simulink model "RCmodel"  (Simulink 7.0)
settings: Solver=ode3  StartTime=0.0  StopTime=0.02  RelTol=1e-3
InitFcn:
  | init;
values from neighbouring files (symbols this model uses):
  C = 1e-6    (= 1e-06)    [initRC.m]
  R = 1000    [initRC.m]
  T0 = tau/5    (= 0.0002)    [initRC.m]
  tau = R*C    (= 0.001)    [initRC.m]
settings Model: Creator=ageorgip  LastModifiedBy=ageorgip

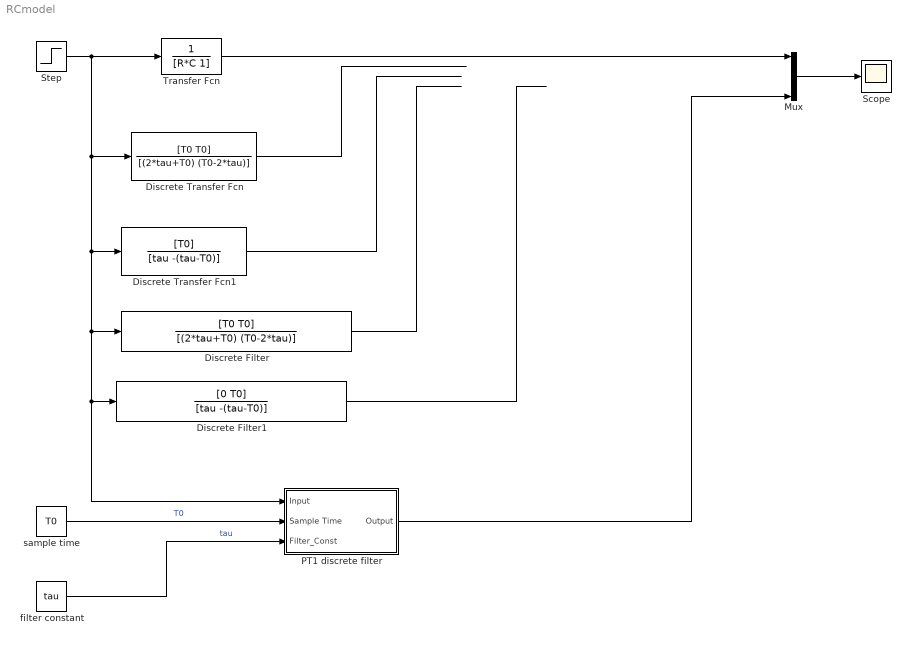
== system RCmodel ==
  Discrete Transfer Fcn : DiscreteTransferFcn  Numerator=[T0 T0]  Denominator=[(2*tau+T0) (T0-2*tau)]  SampleTime=T0
  Discrete Transfer Fcn1 : DiscreteTransferFcn  Numerator=[T0]  Denominator=[tau -(tau-T0)]  SampleTime=T0
  Discrete Filter : DiscreteFilter  Numerator=[T0 T0]  Denominator=[(2*tau+T0) (T0-2*tau)]  SampleTime=T0
  Discrete Filter1 : DiscreteFilter  Numerator=[0 T0]  Denominator=[tau -(tau-T0)]  SampleTime=T0
  Mux : Mux  Inputs=5
  PT1 discrete filter : Subsystem
  Scope : Scope
  Step : Step  Time=0  After=100
  Transfer Fcn : TransferFcn  Denominator=[R*C 1]
  filter constant : Constant  Value=tau  OutDataType=sfix(16)  OutScaling=2^0
  sample time : Constant  Value=T0  OutDataType=sfix(16)  OutScaling=2^0
  wires:
  Step/1 -> Transfer Fcn/1, Discrete Transfer Fcn/1, Discrete Transfer Fcn1/1, Discrete Filter/1, Discrete Filter1/1, PT1 discrete filter/1(Input)
  Transfer Fcn/1 -> Mux/1
  Mux/1 -> Scope/1
  Discrete Transfer Fcn/1 -> ?
  Discrete Transfer Fcn1/1 -> ?
  Discrete Filter/1 -> ?
  Discrete Filter1/1 -> ?
  PT1 discrete filter/1(Output) -> Mux/5
  sample time/1 -> PT1 discrete filter/2(Sample Time)  "T0"
  filter constant/1 -> PT1 discrete filter/3(Filter_Const)  "tau"

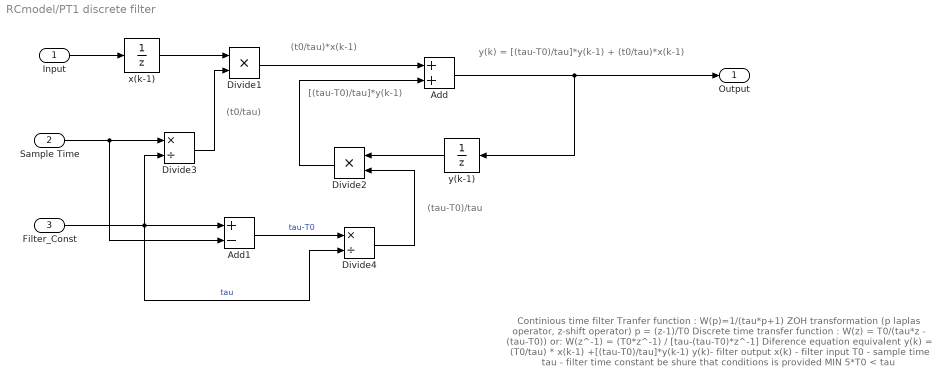
== system RCmodel/PT1 discrete filter ==
  note: (tau-T0)/tau
  note: [(tau-T0)/tau]*y(k-1)
  note: (t0/tau)
  note: (t0/tau)*x(k-1)
  note: y(k) = [(tau-T0)/tau]*y(k-1) + (t0/tau)*x(k-1)
  note: Continious time filter Tranfer function : W(p)=1/(tau*p+1)
      | ZOH transformation (p laplas operator, z-shift operator)
      | p = (z-1)/T0
      | Discrete time transfer function :
      | W(z) = T0/(tau*z - (tau-T0))
      | or: W(z^-1) = (T0*z^-1) / [tau-(tau-T0)*z^-1]
      | Diference equation equivalent
      |  y(k) = (T0/tau) * x(k-1) +[(tau-T0)/tau]*y(k-1)
      | y(k)- filter output
      | x(k) - filter input
      | T0 - sample time
      | tau - filter time constant
      | be shure that conditions is provided MIN  5*T0 < tau
  Input : Inport
  Sample Time : Inport  Port=2
  Filter_Const : Inport  Port=3
  Add : Sum  OutDataType=sfix(16)  OutScaling=2^-10
  Add1 : Sum  Inputs=+-  OutDataType=sfix(16)  OutScaling=2^-10
  Divide1 : Product  Inputs=**  OutDataType=sfix(16)  OutScaling=2^-10
  Divide2 : Product  Orientation=left  Inputs=**  OutDataType=sfix(16)  OutScaling=2^-10
  Divide3 : Product  Inputs=*/  OutDataType=sfix(16)  OutScaling=2^-10
  Divide4 : Product  Inputs=*/  OutDataType=sfix(16)  OutScaling=2^-10
  x(k-1) : UnitDelay  SampleTime=-1
  y(k-1) : UnitDelay  Orientation=left  SampleTime=-1
  Output : Outport
  wires:
  x(k-1)/1 -> Divide1/1
  Divide1/1 -> Add/1
  Add/1 -> y(k-1)/1, Output/1
  y(k-1)/1 -> Divide2/1
  Divide2/1 -> Add/2
  Sample Time/1 -> Add1/2, Divide3/1
  Filter_Const/1 -> Divide4/2, Add1/1, Divide3/2  "tau"
  Divide3/1 -> Divide1/2
  Add1/1 -> Divide4/1  "tau-T0"
  Divide4/1 -> Divide2/2
  Input/1 -> x(k-1)/1
